simulink model "Suspension_tractor_V1_2016a"  (R2016a)
settings: Solver=VariableStepAuto  SolverMode=SingleTasking  StartTime=0.0  StopTime=92  RelTol=1e-3
undefined symbols (not defined in the file): dc, ks, m
settings Model: Creator=mm395  LastModifiedBy=mm395
settings DebuggingCC: SFUnexpectedBacktrackingDiag=error  SFNoUnconditionalDefaultTransitionDiag=error
settings GRTTargetCC: TargetLangStandard=C99 (ISO)  GeneratePreprocessorConditionals=Use local settings
settings ConfigComp: CovMetricSettings=dwe  CovHtmlReporting=off  CovSaveCumulativeToWorkspaceVar=off  CovSaveSingleToWorkspaceVar=off  CovExternalEMLEnable=on

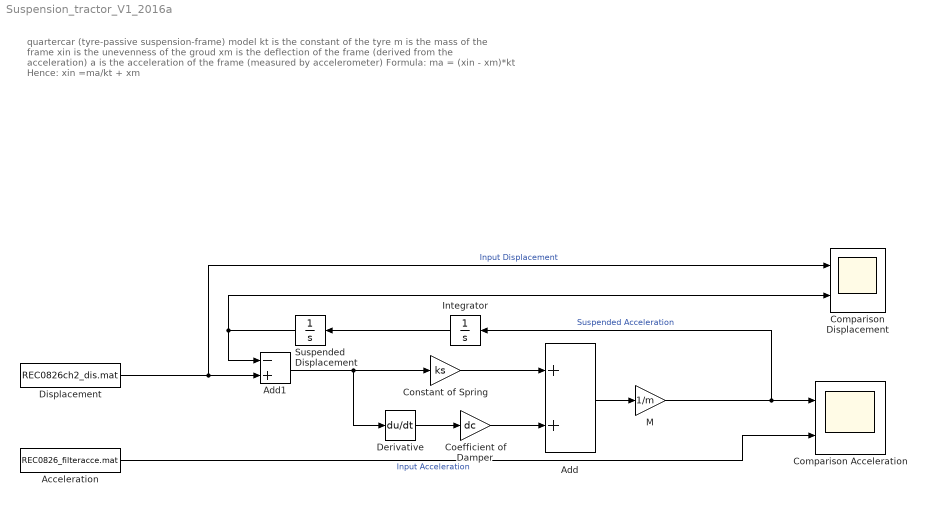
== system Suspension_tractor_V1_2016a ==
  note: quartercar (tyre-passive suspension-frame) model
      | kt is the constant of the tyre
      | m is the mass of the frame
      | xin is the unevenness of the groud
      | xm is the deflection of the frame (derived from the acceleration)
      | a is the acceleration of the frame (measured by accelerometer)
      |
      | Formula: ma = (xin - xm)*kt
      | Hence: xin =ma/kt + xm
  Acceleration : FromFile  FileName=REC0826_filteracce.mat  SampleTime=1/3200  ExtrapolationBeforeFirstDataPoint=Hold first value  ExtrapolationAfterLastDataPoint=Hold last value
  Add : Sum
  Add1 : Sum  Inputs=-+
  Coefficient of Damper : Gain  Gain=dc
  Comparison Acceleration : Scope  NumInputPorts=2
  Comparison Displacement : Scope  NumInputPorts=2
  Constant of Spring : Gain  Gain=ks
  Derivative : Derivative  CoefficientInTFapproximation=0
  Displacement : FromFile  FileName=REC0826ch2_dis.mat  SampleTime=1/3200  ExtrapolationBeforeFirstDataPoint=Hold first value  ExtrapolationAfterLastDataPoint=Hold last value
  Integrator : Integrator
  M : Gain  Gain=1/m
  Suspended Displacement : Integrator
  wires:
  Integrator/1 -> Suspended Displacement/1
  Suspended Displacement/1 -> Comparison Displacement/2, Add1/1
  Derivative/1 -> Coefficient of Damper/1
  Acceleration/1 -> Comparison Acceleration/2  "Input Acceleration"
  Add1/1 -> Derivative/1, Constant of Spring/1
  Constant of Spring/1 -> Add/1
  Displacement/1 -> Add1/2, Comparison Displacement/1  "Input Displacement"
  M/1 -> Comparison Acceleration/1, Integrator/1  "Suspended Acceleration"
  Add/1 -> M/1
  Coefficient of Damper/1 -> Add/2
